simulink model "muc2tn2dknc"  (R2015a)
settings: Solver=ode45  StartTime=0.0  StopTime=10  RelTol=1e-3
settings Model: Creator=nguye  LastModifiedBy=nguye

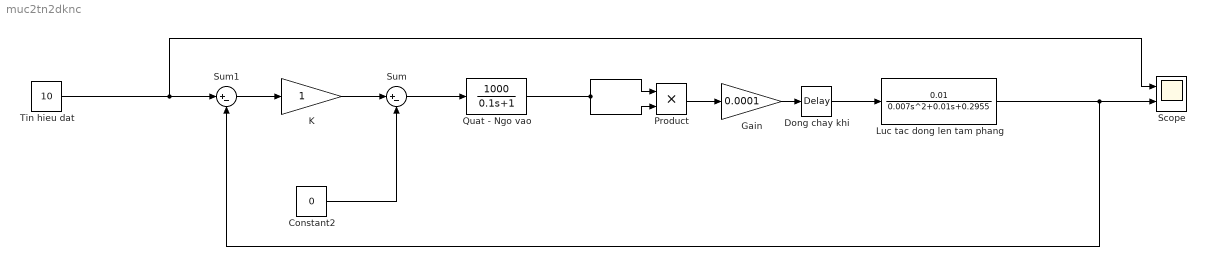
== system muc2tn2dknc ==
  Constant2 : Constant  Value=0
  Dong chay khi : TransportDelay  DelayTime=0.02
  Gain : Gain  Gain=0.0001
  K : Gain
  Luc tac dong len tam phang : TransferFcn  Numerator=[0.01]  Denominator=[0.007 0.01 0.2955]
  Product : Product
  Quat - Ngo vao : TransferFcn  Numerator=[1000]  Denominator=[0.1 1]
  Scope : Scope  NumInputPorts=2
      settings: YMin=-5~-5  YMax=5~5
  Sum : Sum  Inputs=|+-
  Sum1 : Sum  Inputs=|+-
  Tin hieu dat : Constant  Value=10
  wires:
  Sum/1 -> Quat - Ngo vao/1
  Product/1 -> Gain/1
  Gain/1 -> Dong chay khi/1
  Dong chay khi/1 -> Luc tac dong len tam phang/1
  Quat - Ngo vao/1 -> Product/2, Product/1
  Constant2/1 -> Sum/2
  K/1 -> Sum/1
  Tin hieu dat/1 -> Scope/1, Sum1/1
  Sum1/1 -> K/1
  Luc tac dong len tam phang/1 -> Sum1/2, Scope/2
